simulink model "ex4"  (R2020a)
settings: Solver=VariableStepAuto  StartTime=0.0  StopTime=10.0  RelTol=1e-3

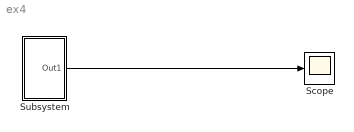
== system ex4 ==
  Scope : Scope
  Subsystem : Subsystem  mask{Te=0}
      mask prompts: Te "Te="
  wires:
  Subsystem/1(Out1) -> Scope/1

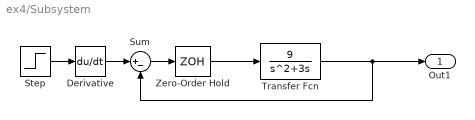
== system ex4/Subsystem ==
  Derivative : Derivative
  Step : Step  SampleTime=Te
  Sum : Sum  Inputs=|+-  SampleTime=Te
  Transfer Fcn : TransferFcn  Numerator=[9]  Denominator=[1 3 0]
  Zero-Order Hold : ZeroOrderHold  SampleTime=-1
  Out1 : Outport
  wires:
  Derivative/1 -> Sum/1
  Transfer Fcn/1 -> Out1/1, Sum/2
  Step/1 -> Derivative/1
  Zero-Order Hold/1 -> Transfer Fcn/1
  Sum/1 -> Zero-Order Hold/1
